simulink model "PMSM_FOC_Basic_v2"  (R2024a)
settings: Solver=FixedStepDiscrete  StartTime=0.0  StopTime=1.2  FixedStep=1e-4  RelTol=1e-3
Description:
  | Runnable basic PMSM FOC model: 100 us current loop, 1 ms speed loop, SVPWM average inverter, discrete PMSM plant.
settings Model: Creator=18283  LastModifiedBy=18283
settings DataIOCC: SaveOutput=off  SignalLogging=off  SaveTime=off

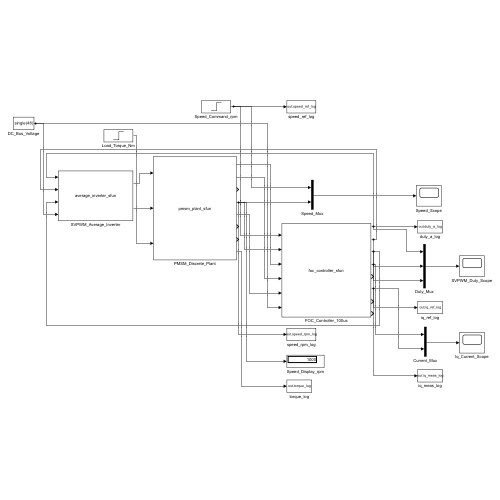
[thumbnail: Simulink's stored preview of the top-level diagram]
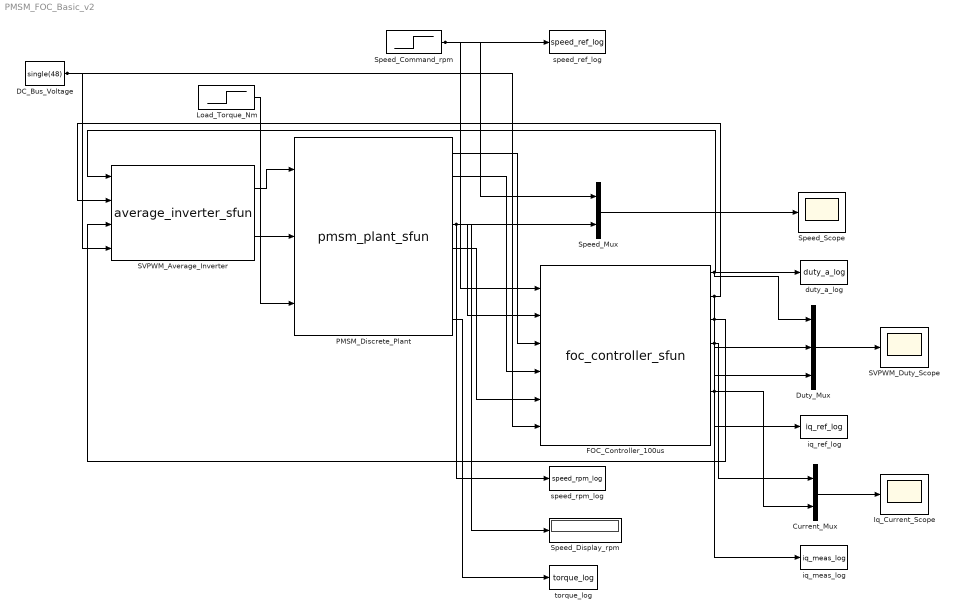
== system PMSM_FOC_Basic_v2 ==
  Current_Mux : Mux  Inputs=2
  DC_Bus_Voltage : Constant  Value=single(48)  OutDataTypeStr=single  SampleTime=1e-4
  Duty_Mux : Mux  Inputs=3
  FOC_Controller_100us : M-S-Function  FunctionName=foc_controller_sfun
  Iq_Current_Scope : Scope
  Load_Torque_Nm : Step  Time=0.50  After=0.20  OutDataTypeStr=single  SampleTime=1e-4
  PMSM_Discrete_Plant : M-S-Function  FunctionName=pmsm_plant_sfun
  SVPWM_Average_Inverter : M-S-Function  FunctionName=average_inverter_sfun
  SVPWM_Duty_Scope : Scope
  Speed_Command_rpm : Step  Time=0.05  After=1000  OutDataTypeStr=single  SampleTime=1e-4
  Speed_Display_rpm : Display
  Speed_Mux : Mux  Inputs=2
  Speed_Scope : Scope
  duty_a_log : ToWorkspace  VariableName=duty_a_log  SaveFormat=Timeseries  SampleTime=-1
  iq_meas_log : ToWorkspace  VariableName=iq_meas_log  SaveFormat=Timeseries  SampleTime=-1
  iq_ref_log : ToWorkspace  VariableName=iq_ref_log  SaveFormat=Timeseries  SampleTime=-1
  speed_ref_log : ToWorkspace  VariableName=speed_ref_log  SaveFormat=Timeseries  SampleTime=-1
  speed_rpm_log : ToWorkspace  VariableName=speed_rpm_log  SaveFormat=Timeseries  SampleTime=-1
  torque_log : ToWorkspace  VariableName=torque_log  SaveFormat=Timeseries  SampleTime=-1
  wires:
  DC_Bus_Voltage/1 -> FOC_Controller_100us/6, SVPWM_Average_Inverter/4
  Load_Torque_Nm/1 -> PMSM_Discrete_Plant/3
  SVPWM_Average_Inverter/1 -> PMSM_Discrete_Plant/1
  SVPWM_Average_Inverter/2 -> PMSM_Discrete_Plant/2
  Speed_Command_rpm/1 -> Speed_Mux/1, FOC_Controller_100us/1, speed_ref_log/1
  PMSM_Discrete_Plant/4 -> FOC_Controller_100us/2, Speed_Mux/2, Speed_Display_rpm/1, speed_rpm_log/1
  PMSM_Discrete_Plant/2 -> FOC_Controller_100us/4
  PMSM_Discrete_Plant/1 -> FOC_Controller_100us/3
  PMSM_Discrete_Plant/5 -> FOC_Controller_100us/5
  FOC_Controller_100us/4 -> Current_Mux/1, iq_ref_log/1
  PMSM_Discrete_Plant/8 -> torque_log/1
  Speed_Mux/1 -> Speed_Scope/1
  FOC_Controller_100us/1 -> SVPWM_Average_Inverter/1, Duty_Mux/1, duty_a_log/1
  FOC_Controller_100us/2 -> Duty_Mux/2, SVPWM_Average_Inverter/2
  FOC_Controller_100us/3 -> SVPWM_Average_Inverter/3, Duty_Mux/3
  FOC_Controller_100us/6 -> iq_meas_log/1, Current_Mux/2
  Duty_Mux/1 -> SVPWM_Duty_Scope/1
  Current_Mux/1 -> Iq_Current_Scope/1
